simulink model "Comunicacao_Simulink_R2018b"  (R2018b)
settings: Solver=VariableStepAuto  StartTime=0.0  StopTime=33  RelTol=1e-3
libraries: dspsrcs4 x2, commsynccomp2 x1, simulink x1, commfilt2 x1, commutil2 x1
settings Model: Creator=rafae  LastModifiedBy=rafae

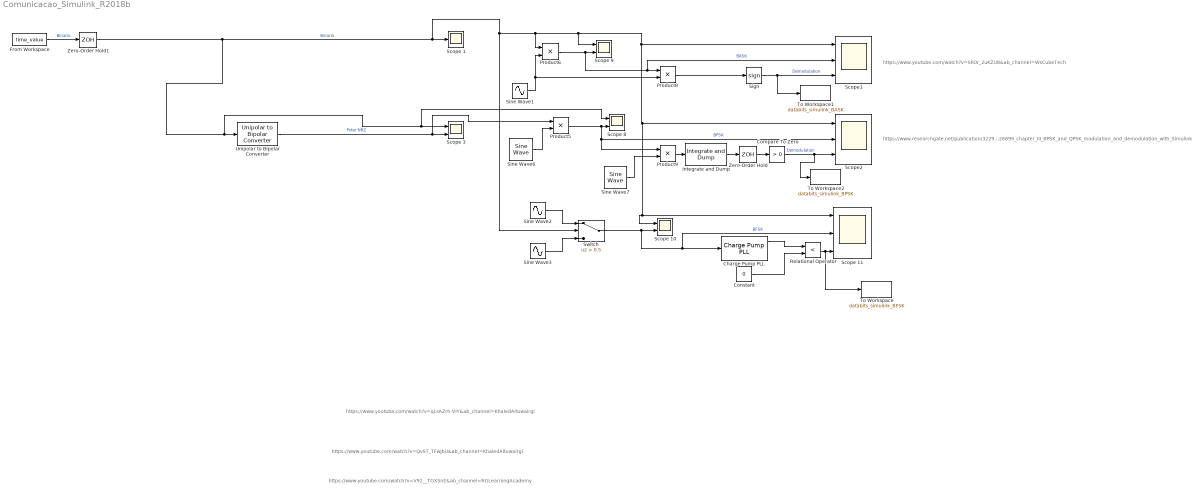
== system Comunicacao_Simulink_R2018b ==
  note: https://www.researchgate.net/publication/322926899_chapter_III_BPSK_and_QPSK_modulation_and_demodulation_with_Simulink
  note: https://www.youtube.com/watch?v=SR0r_2uKZU8&ab_channel=WsCubeTech
  note: https://www.youtube.com/watch?v=qLsAZrh-VIY&ab_channel=KhaledAltuwairgi
  note: https://www.youtube.com/watch?v=V92__TGXSnE&ab_channel=RGLearningAcademy
  note: https://www.youtube.com/watch?v=QvST_TFwJbU&ab_channel=KhaledAltuwairgi
  Charge Pump PLL : commsynccomp2/Charge Pump PLL  Fn=[2*pi*1]  Fd=[1 2*pi*1]  Kvco=4  Fc=10  Ph=0  Ac=1
      settings: SourceProductName=Communications Toolbox  SourceProductBaseCode=CM
  Compare To Zero : simulink/Logic and Bit Operations/Compare To Zero  relop=>  OutDataTypeStr=boolean
  Constant : Constant  Value=0
  From Workspace : FromWorkspace  VariableName=time_value  SampleTime=0
  Integrate and Dump : commfilt2/Integrate and Dump  obssamples=100  offsetsamples=0  nodump=on  roundingMode=Floor  overflowMode=off  outputDataTypeStr=Inherit: Same as accumulator  outputLastDataTypeStr=Inherit: Same as accumulator
      settings: SourceProductName=Communications Toolbox
  Product{5..6,8..9} (4 alike) : Product
  Relational Operator : RelationalOperator  Operator=<  OutDataTypeStr=boolean  RndMeth=Simplest
  Scope 1 : Scope
  Scope {3,8..10} (4 alike) : Scope  NumInputPorts=2
  Scope 11 : Scope  NumInputPorts=3
  Scope1 : Scope  NumInputPorts=3
  Scope2 : Scope  NumInputPorts=3
  Sign : Signum
  Sine Wave1 : Sin  Frequency=2*pi*2  SampleTime=0
  Sine Wave2 : Sin  Frequency=2*pi*4  SampleTime=0
  Sine Wave3 : Sin  Frequency=2*pi*12  SampleTime=0
  Sine Wave6 : dspsrcs4/Sine Wave  Amplitude=1  Frequency=5  Phase=0  SampleMode=Discrete  OutComplex=Real  CompMethod=Trigonometric fcn  TableSize=Speed  SampleTime=1/1000  SamplesPerFrame=1  ResetState=Restart at time zero  OutputFrames=off  dataType=double  wordLen=16  udDataType=sfix(16)  fracBitsMode=Best precision  numFracBits=15  OutDataTypeStr=double  LastOutDataTypeStr=double
  Sine Wave7 : dspsrcs4/Sine Wave  Amplitude=1  Frequency=5  Phase=0  SampleMode=Discrete  OutComplex=Real  CompMethod=Trigonometric fcn  TableSize=Speed  SampleTime=1/1000  SamplesPerFrame=1  ResetState=Restart at time zero  OutputFrames=off  dataType=double  wordLen=16  udDataType=sfix(16)  fracBitsMode=Best precision  numFracBits=15  OutDataTypeStr=double  LastOutDataTypeStr=double
  Switch : Switch  Criteria=u2 > Threshold  Threshold=0.5
  To Workspace : ToWorkspace  VariableName=databits_simulink_BFSK  SaveFormat=Timeseries  SampleTime=-1
  To Workspace1 : ToWorkspace  VariableName=databits_simulink_BASK  SaveFormat=Timeseries  SampleTime=-1
  To Workspace2 : ToWorkspace  VariableName=databits_simulink_BPSK  SaveFormat=Timeseries  SampleTime=-1
  Unipolar to Bipolar Converter : commutil2/Unipolar to Bipolar Converter  M=2  polarity=Positive  dataType=Inherit via internal rule
      settings: SourceProductName=Communications Toolbox
  Zero-Order Hold : ZeroOrderHold  SampleTime=-1
  Zero-Order Hold1 : ZeroOrderHold  SampleTime=-1
  wires:
  Zero-Order Hold1/1 -> Switch/2, Scope2/1, Scope 10/1, Scope 11/1, Scope1/1, Scope 9/1, Product6/1, Scope 1/1, Scope 8/1, Scope 3/1, Unipolar to Bipolar Converter/1  "Binario"
  Unipolar to Bipolar Converter/1 -> Product5/1, Scope 3/2  "Polar NRZ"
  Sine Wave1/1 -> Product6/2, Product8/2
  Product5/1 -> Product9/1, Scope2/2, Scope 8/2  "BPSK"
  Product6/1 -> Product8/1, Scope1/2, Scope 9/2  "BASK"
  Switch/1 -> Scope 10/2, Scope 11/2, Charge Pump PLL/1  "BFSK"
  Sine Wave2/1 -> Switch/1
  Sine Wave3/1 -> Switch/3
  Constant/1 -> Relational Operator/2
  Charge Pump PLL/1 -> Relational Operator/1
  Relational Operator/1 -> To Workspace/1, Scope 11/3
  Product8/1 -> Sign/1
  Sign/1 -> To Workspace1/1, Scope1/3  "Demodulation"
  Product9/1 -> Integrate and Dump/1
  Integrate and Dump/1 -> Zero-Order Hold/1
  Zero-Order Hold/1 -> Compare To Zero/1
  Compare To Zero/1 -> To Workspace2/1, Scope2/3  "Demodulation"
  Sine Wave7/1 -> Product9/2
  Sine Wave6/1 -> Product5/2
  From Workspace/1 -> Zero-Order Hold1/1  "Binario"
